simulink model "simuMotorFeedforward2"  (R2014a)
settings: Solver=ode45  StartTime=0.0  StopTime=3  MaxStep=0.0001  RelTol=1e-3
values from neighbouring files (symbols this model uses):
  contr = param    [parametres.m]
undefined symbols (not defined in the file or in its folder): param
settings Model: Creator=Etienne  LastModifiedBy=Etienne

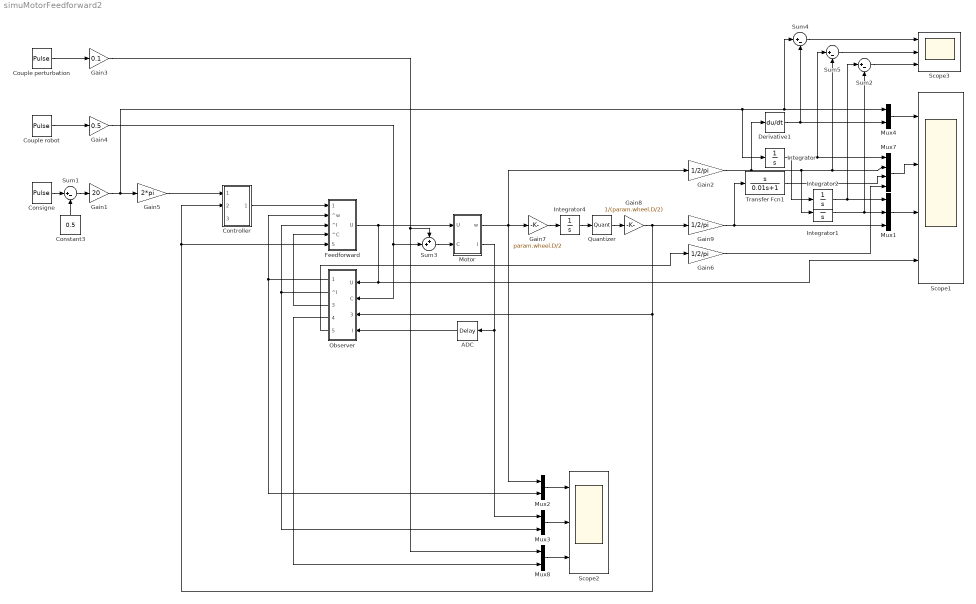
== system simuMotorFeedforward2 ==
  ADC : TransportDelay  DelayTime=param.adc.retard
  Consigne : DiscretePulseGenerator  PulseType=Time based  Period=1  PulseWidth=50  PhaseDelay=0.25/2
  Constant3 : Constant  Value=0.5
  Controller : Subsystem
  Couple perturbation : DiscretePulseGenerator  PulseType=Time based  Period=2/3  PulseWidth=50  PhaseDelay=0.3
  Couple robot : DiscretePulseGenerator  PulseType=Time based  Period=1.5  PulseWidth=50  PhaseDelay=0.1
  Derivative1 : Derivative
  Feedforward : Subsystem
  Gain1 : Gain  Gain=20
  Gain2 : Gain  Gain=1/2/pi
  Gain3 : Gain  Gain=0.1
  Gain4 : Gain  Gain=0.5
  Gain5 : Gain  Gain=2*pi
  Gain6 : Gain  Gain=1/2/pi
  Gain7 : Gain  Gain=param.wheel.D/2
  Gain8 : Gain  Gain=1/(param.wheel.D/2)
  Gain9 : Gain  Gain=1/2/pi
  Integrator{,1..2,4} (4 alike) : Integrator
  Motor : Subsystem
  Mux1 : Mux  Inputs=3
  Mux{2..4,8} (4 alike) : Mux  Inputs=2
  Mux7 : Mux
  Observer : Subsystem
  Quantizer : Quantizer  QuantizationInterval=param.codeur.resolution
  Scope1 : Scope  NumInputPorts=4
      settings: TimeRange=3  YMin=-60~-2~-0.5~-10  YMax=60~4~4~25  SaveName=ScopeData2  MaxDataPoints=500000
  Scope2 : Scope  NumInputPorts=3
      settings: TimeRange=3  YMin=-10~-3~-0.04  YMax=25~5~0.1  MaxDataPoints=500000
  Scope3 : Scope  NumInputPorts=3
      settings: TimeRange=3  YMin=-80~-0.15~-0.0006000000000000001  YMax=80~0.09999999999999998~0.0014  SaveName=ScopeData3  MaxDataPoints=500000
  Sum{1..2,4..5} (4 alike) : Sum  Inputs=|+-
  Sum3 : Sum  Inputs=++|
  Transfer Fcn1 : TransferFcn  Numerator=[1 0]  Denominator=[0.01 1]
  wires:
  Couple perturbation/1 -> Gain3/1
  Motor/2(I) -> Mux3/1, ADC/1
  Consigne/1 -> Sum1/1
  Sum1/1 -> Gain1/1
  Constant3/1 -> Sum1/2
  Gain2/1 -> Derivative1/1, Mux7/2, Sum5/2, Integrator1/1
  Feedforward/1(U) -> Motor/1(U), Scope1/4, Observer/1(U)
  ADC/1 -> Observer/4(I)
  Mux4/1 -> Scope1/1
  Observer/1(^w) -> Mux2/2, Feedforward/2(^w)
  Observer/2(^I) -> Feedforward/3(^I), Mux3/2
  Observer/3(^C) -> Feedforward/4(^C)
  Gain1/1 -> Gain5/1, Integrator/1, Mux4/1, Sum4/1
  Gain3/1 -> Sum3/1, Mux8/1
  Derivative1/1 -> Mux4/2, Sum4/2
  Mux7/1 -> Scope1/2
  Integrator/1 -> Mux7/1, Sum5/1, Integrator2/1
  Sum4/1 -> Scope3/1
  Sum5/1 -> Scope3/2
  Mux1/1 -> Scope1/3
  Integrator1/1 -> Mux1/2, Sum2/2
  Integrator2/1 -> Mux1/1, Sum2/1
  Sum2/1 -> Scope3/3
  Gain4/1 -> Sum3/2, Observer/2(C)
  Integrator4/1 -> Quantizer/1
  Quantizer/1 -> Gain8/1
  Gain9/1 -> Transfer Fcn1/1, Mux1/3
  Motor/1(w) -> Gain7/1, Gain2/1, Mux2/1
  Gain7/1 -> Integrator4/1
  Mux2/1 -> Scope2/1
  Mux3/1 -> Scope2/2
  Mux8/1 -> Scope2/3
  Gain8/1 -> Observer/3(teta), Feedforward/5(teta), Controller/2(teta), Gain9/1
  Gain5/1 -> Controller/1(cons)
  Sum3/1 -> Motor/2(C)
  Couple robot/1 -> Gain4/1
  Controller/1(out) -> Feedforward/1(cons)
  Observer/4(Cerr) -> Mux8/2
  Transfer Fcn1/1 -> Mux7/3
  Gain6/1 -> Mux7/4
  Observer/5(^w1) -> Gain6/1

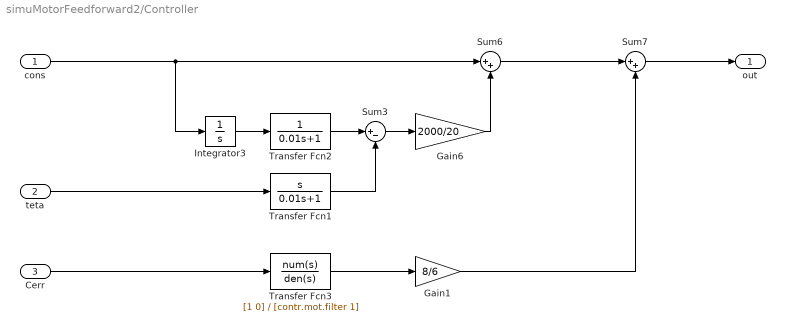
== system simuMotorFeedforward2/Controller ==
  cons : Inport
  teta : Inport  Port=2
  Cerr : Inport  Port=3
  Gain1 : Gain  Gain=8/6
  Gain6 : Gain  Gain=2000/20
  Integrator3 : Integrator
  Sum3 : Sum  Inputs=|+-
  Sum6 : Sum  Inputs=|++
  Sum7 : Sum  Inputs=|++
  Transfer Fcn1 : TransferFcn  Numerator=[1 0]  Denominator=[0.01 1]
  Transfer Fcn2 : TransferFcn  Denominator=[0.01 1]
  Transfer Fcn3 : TransferFcn  Numerator=[1 0]  Denominator=[contr.mot.filter 1]
  out : Outport
  wires:
  Transfer Fcn2/1 -> Sum3/1
  teta/1 -> Transfer Fcn1/1
  Integrator3/1 -> Transfer Fcn2/1
  cons/1 -> Sum6/1, Integrator3/1
  Sum3/1 -> Gain6/1
  Gain1/1 -> Sum7/2
  Sum7/1 -> out/1
  Sum6/1 -> Sum7/1
  Gain6/1 -> Sum6/2
  Transfer Fcn1/1 -> Sum3/2
  Transfer Fcn3/1 -> Gain1/1
  Cerr/1 -> Transfer Fcn3/1

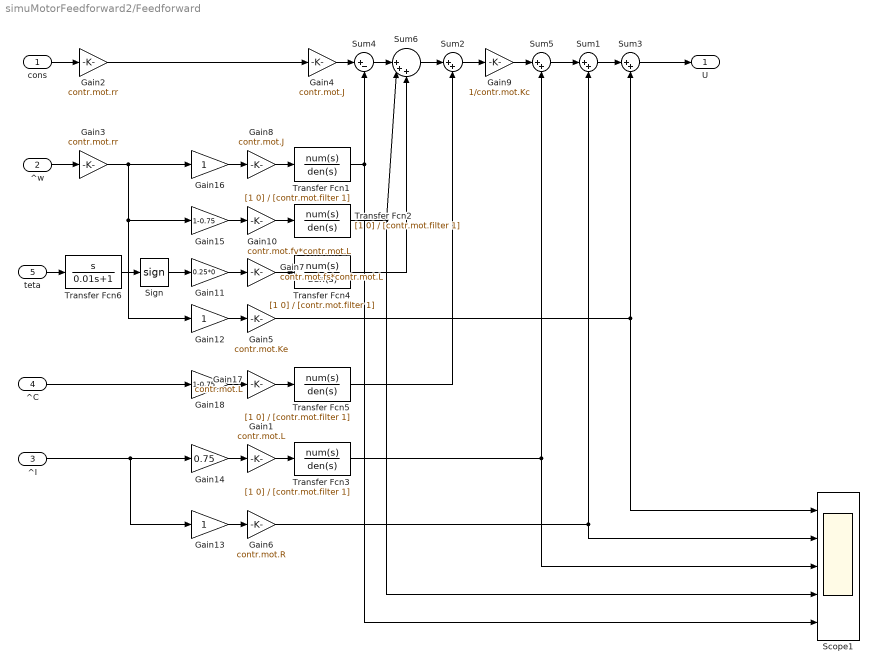
== system simuMotorFeedforward2/Feedforward ==
  cons : Inport
  ^w : Inport  Port=2
  ^I : Inport  Port=3
  ^C : Inport  Port=4
  teta : Inport  Port=5
  Gain1 : Gain  Gain=contr.mot.L
  Gain10 : Gain  Gain=contr.mot.fv*contr.mot.L
  Gain11 : Gain  Gain=0.25*0
  Gain12 : Gain
  Gain13 : Gain
  Gain14 : Gain  Gain=0.75
  Gain15 : Gain  Gain=1-0.75
  Gain16 : Gain
  Gain17 : Gain  Gain=contr.mot.L
  Gain18 : Gain  Gain=1-0.75
  Gain2 : Gain  Gain=contr.mot.rr
  Gain3 : Gain  Gain=contr.mot.rr
  Gain4 : Gain  Gain=contr.mot.J
  Gain5 : Gain  Gain=contr.mot.Ke
  Gain6 : Gain  Gain=contr.mot.R
  Gain7 : Gain  Gain=contr.mot.fs*contr.mot.L
  Gain8 : Gain  Gain=contr.mot.J
  Gain9 : Gain  Gain=1/contr.mot.Kc
  Scope1 : Scope  NumInputPorts=5
      settings: TimeRange=3  YMin=-5~-10~-15000~-0.03~-15  YMax=15~10~15000~0.03~15  MaxDataPoints=500000
  Sign : Signum  ZeroCross=off
  Sum{1..3,5} (4 alike) : Sum  Inputs=|++
  Sum4 : Sum  Inputs=|+-
  Sum6 : Sum  Inputs=||+++
  Transfer Fcn{1..5} (5 alike) : TransferFcn  Numerator=[1 0]  Denominator=[contr.mot.filter 1]
  Transfer Fcn6 : TransferFcn  Numerator=[1 0]  Denominator=[0.01 1]
  U : Outport
  wires:
  Gain5/1 -> Sum3/2, Scope1/1
  Gain8/1 -> Transfer Fcn1/1
  Gain3/1 -> Gain16/1, Gain15/1, Gain12/1
  Gain2/1 -> Gain4/1
  Sum1/1 -> Sum3/1
  Gain6/1 -> Sum1/2, Scope1/2
  Sum3/1 -> U/1
  Transfer Fcn1/1 -> Scope1/5, Sum4/2
  Transfer Fcn3/1 -> Sum5/2, Scope1/3
  Sum5/1 -> Sum1/1
  Gain12/1 -> Gain5/1
  Gain9/1 -> Sum5/1
  Gain1/1 -> Transfer Fcn3/1
  Gain15/1 -> Gain10/1
  Gain16/1 -> Gain8/1
  Gain13/1 -> Gain6/1
  Gain14/1 -> Gain1/1
  Sum4/1 -> Sum6/1
  cons/1 -> Gain2/1
  ^w/1 -> Gain3/1
  ^I/1 -> Gain14/1, Gain13/1
  Gain4/1 -> Sum4/1
  Gain10/1 -> Transfer Fcn2/1
  Transfer Fcn2/1 -> Sum6/2, Scope1/4
  Gain7/1 -> Transfer Fcn4/1
  Gain11/1 -> Gain7/1
  Sign/1 -> Gain11/1
  Transfer Fcn4/1 -> Sum6/3
  Gain17/1 -> Transfer Fcn5/1
  Gain18/1 -> Gain17/1
  Sum6/1 -> Sum2/1
  Sum2/1 -> Gain9/1
  Transfer Fcn5/1 -> Sum2/2
  ^C/1 -> Gain18/1
  teta/1 -> Transfer Fcn6/1
  Transfer Fcn6/1 -> Sign/1

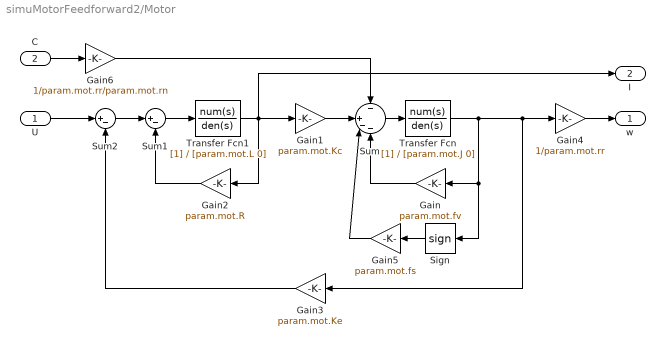
== system simuMotorFeedforward2/Motor ==
  U : Inport
  C : Inport  Port=2
  Gain : Gain  Gain=param.mot.fv
  Gain1 : Gain  Gain=param.mot.Kc
  Gain2 : Gain  Gain=param.mot.R
  Gain3 : Gain  Gain=param.mot.Ke
  Gain4 : Gain  Gain=1/param.mot.rr
  Gain5 : Gain  Gain=param.mot.fs
  Gain6 : Gain  Gain=1/param.mot.rr/param.mot.rn
  Sign : Signum  ZeroCross=off
  Sum : Sum  Inputs=-|+--
  Sum1 : Sum  Inputs=|+-
  Sum2 : Sum  Inputs=|+-
  Transfer Fcn : TransferFcn  Denominator=[param.mot.J 0]
  Transfer Fcn1 : TransferFcn  Denominator=[param.mot.L 0]
  w : Outport
  I : Outport  Port=2
  wires:
  Gain1/1 -> Sum/2
  Transfer Fcn/1 -> Gain3/1, Gain4/1, Sign/1, Gain/1
  Gain3/1 -> Sum2/2
  Sum2/1 -> Sum1/1
  Gain2/1 -> Sum1/2
  Sum1/1 -> Transfer Fcn1/1
  U/1 -> Sum2/1
  C/1 -> Gain6/1
  Gain6/1 -> Sum/1
  Gain4/1 -> w/1
  Sum/1 -> Transfer Fcn/1
  Transfer Fcn1/1 -> Gain1/1, I/1, Gain2/1
  Sign/1 -> Gain5/1
  Gain/1 -> Sum/4
  Gain5/1 -> Sum/3

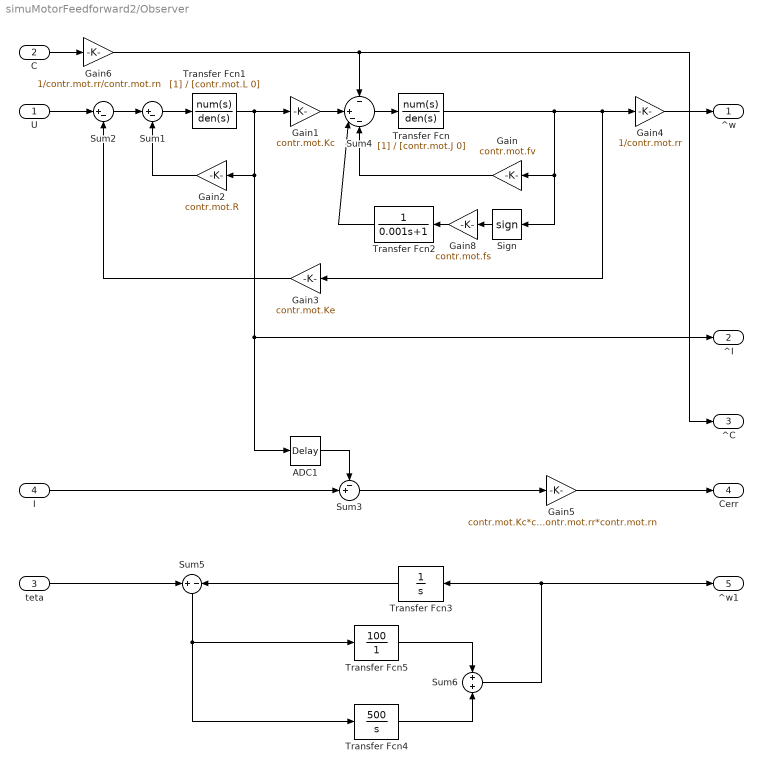
== system simuMotorFeedforward2/Observer ==
  U : Inport
  C : Inport  Port=2
  teta : Inport  Port=3
  I : Inport  Port=4
  ADC1 : TransportDelay  DelayTime=contr.adc.retard
  Gain : Gain  Gain=contr.mot.fv
  Gain1 : Gain  Gain=contr.mot.Kc
  Gain2 : Gain  Gain=contr.mot.R
  Gain3 : Gain  Gain=contr.mot.Ke
  Gain4 : Gain  Gain=1/contr.mot.rr
  Gain5 : Gain  Gain=contr.mot.Kc*contr.mot.rr*contr.mot.rn
  Gain6 : Gain  Gain=1/contr.mot.rr/contr.mot.rn
  Gain8 : Gain  Gain=contr.mot.fs
  Sign : Signum  ZeroCross=off
  Sum1 : Sum  Inputs=|+-
  Sum2 : Sum  Inputs=|+-
  Sum3 : Sum  Inputs=-+|
  Sum4 : Sum  Inputs=-|+--
  Sum5 : Sum  Inputs=+|-
  Sum6 : Sum
  Transfer Fcn : TransferFcn  Denominator=[contr.mot.J 0]
  Transfer Fcn1 : TransferFcn  Denominator=[contr.mot.L 0]
  Transfer Fcn2 : TransferFcn  Denominator=[0.001 1]
  Transfer Fcn3 : TransferFcn  Denominator=[1 0]
  Transfer Fcn4 : TransferFcn  Numerator=[500]  Denominator=[1 0]
  Transfer Fcn5 : TransferFcn  Numerator=[100]  Denominator=[1]
  ^w : Outport
  ^I : Outport  Port=2
  ^C : Outport  Port=3
  Cerr : Outport  Port=4
  ^w1 : Outport  Port=5
  wires:
  Transfer Fcn/1 -> Gain3/1, Gain4/1, Gain/1, Sign/1
  Gain3/1 -> Sum2/2
  Sum2/1 -> Sum1/1
  Sum1/1 -> Transfer Fcn1/1
  U/1 -> Sum2/1
  C/1 -> Gain6/1
  Transfer Fcn1/1 -> ^I/1, ADC1/1, Gain2/1, Gain1/1
  Sum3/1 -> Gain5/1
  I/1 -> Sum3/2
  ADC1/1 -> Sum3/1
  Gain2/1 -> Sum1/2
  Gain4/1 -> ^w/1
  Sign/1 -> Gain8/1
  Gain/1 -> Sum4/4
  Sum4/1 -> Transfer Fcn/1
  Gain1/1 -> Sum4/2
  Gain8/1 -> Transfer Fcn2/1
  Transfer Fcn2/1 -> Sum4/3
  Gain6/1 -> ^C/1, Sum4/1
  Gain5/1 -> Cerr/1
  teta/1 -> Sum5/1
  Transfer Fcn3/1 -> Sum5/2
  Sum5/1 -> Transfer Fcn5/1, Transfer Fcn4/1
  Sum6/1 -> Transfer Fcn3/1, ^w1/1
  Transfer Fcn4/1 -> Sum6/2
  Transfer Fcn5/1 -> Sum6/1
